simulink model "s1_7"  (R2020b)
settings: Solver=VariableStepAuto  StartTime=0.0  StopTime=20  RelTol=1e-3
values from neighbouring files (symbols this model uses):
  y0 = [1,0.5,0.5,0.2]    [s1_7c.m]
undefined symbols (not defined in the file or in its folder): a, b, c, d
settings Model: Creator=huang  LastModifiedBy=huang

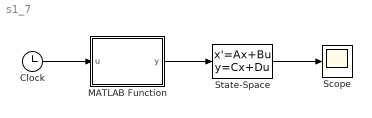
== system s1_7 ==
  Clock : Clock
  MATLAB Function : MATLAB Function  TreatAsAtomicUnit=on
  Scope : Scope
  State-Space : StateSpace  A=a  B=b  C=c  D=d  InitialCondition=y0
  wires:
  Clock/1 -> MATLAB Function/1(u)
  MATLAB Function/1(y) -> State-Space/1
  State-Space/1 -> Scope/1

== matlab function s1_7/MATLAB Function ==
  data: u input; y output
function y = signal(u)
    y=exp(-3*u)+exp(-5*u)*sin(4*u+pi/3);
end
